simulink model "ctrl_simulink"  (R2014a)
settings: Solver=ode45  StartTime=0.0  StopTime=200  RelTol=1e-3
StartFcn:
  | clear all
libraries: simulink x1
settings Model: Creator=John  LastModifiedBy=John

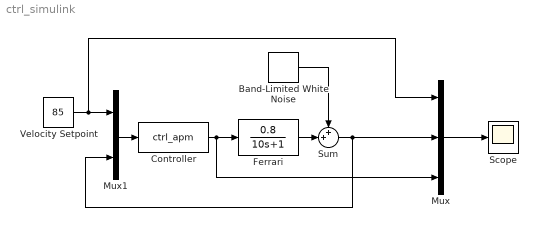
== system ctrl_simulink ==
  Band-Limited White Noise : simulink/Sources/Band-Limited White Noise  Cov=[0.1]  Ts=1  seed=[23341]
  Controller : MATLABFcn  MATLABFcn=ctrl_apm  OutputDimensions=1  SampleTime=1
  Ferrari : TransferFcn  Numerator=[0.8]  Denominator=[10 1]
  Mux : Mux  Inputs=3
  Mux1 : Mux  Inputs=2
  Scope : Scope
      settings: YMin=0  YMax=100
  Sum : Sum  Inputs=++|
  Velocity Setpoint : Constant  Value=85
  wires:
  Controller/1 -> Mux/3, Ferrari/1
  Ferrari/1 -> Sum/2
  Band-Limited White Noise/1 -> Sum/1
  Mux1/1 -> Controller/1
  Sum/1 -> Mux1/2, Mux/2
  Velocity Setpoint/1 -> Mux/1, Mux1/1
  Mux/1 -> Scope/1
